simulink model "LAB2_2"  (R2022a)
settings: Solver=VariableStepAuto  StartTime=0.0  StopTime=10.0  RelTol=1e-3
settings Model: Creator=hyhung3  LastModifiedBy=hyhung3

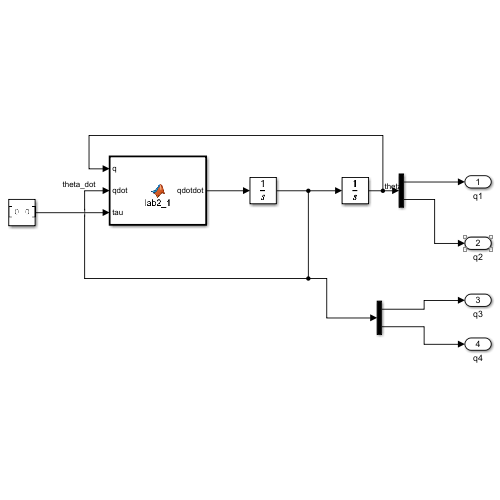
[thumbnail: Simulink's stored preview of the top-level diagram]
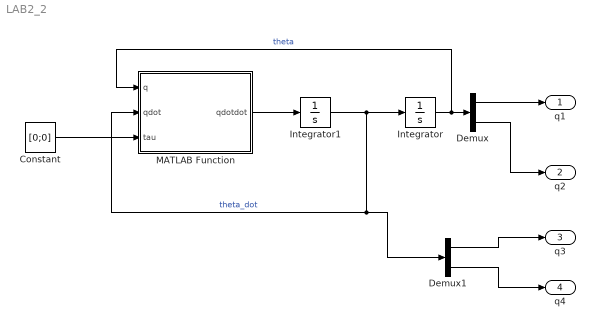
== system LAB2_2 ==
  Constant : Constant  Value=[0;0]
  Demux : Demux  Outputs=2
  Demux1 : Demux  Outputs=2
  Integrator : Integrator  InitialCondition=[0;0]
  Integrator1 : Integrator  InitialCondition=[0;0]
  MATLAB Function : MATLAB Function  TreatAsAtomicUnit=on
  q1 : Outport
  q2 : Outport  Port=2
  q3 : Outport  Port=3
  q4 : Outport  Port=4
  wires:
  Demux/2 -> q2/1
  Demux/1 -> q1/1
  Demux1/1 -> q3/1
  MATLAB Function/1(qdotdot) -> Integrator1/1
  Demux1/2 -> q4/1
  Integrator/1 -> MATLAB Function/1(q), Demux/1  "theta"
  Integrator1/1 -> Integrator/1, Demux1/1, MATLAB Function/2(qdot)  "theta_dot"
  Constant/1 -> MATLAB Function/3(tau)

== matlab function LAB2_2/MATLAB Function ==
  data: q input; qdotdot output; qdot input; tau input
function qdotdot = lab2_1(q,qdot,tau)
g = 9.81;

theta2 = q(1);
theta3 = q(2);

theta2_dot = qdot(1);
theta3_dot = qdot(2);

p = [0.03; 0.0128; 0.0076; 0.0753; 0.0298];

p1 = p(1);
p2 = p(2);
p3 = p(3);
p4 = p(4);
p5 = p(5);

M = [[p1                        -p3*sin(theta3 - theta2)];
     [-p3*sin(theta3 - theta2)                        p2]];
C = [[0                                 -p3*cos(theta3 - theta2)*theta3_dot];
     [p3*cos(theta3 - theta2)*theta2_dot                                  0]];

G = [-p4*g*sin(theta2);
       -p5*g*cos(theta3)];

qdotdot = (inv(M))*tau - (inv(M))*C*qdot - (inv(M))*G;
